simulink model "DVA_P1"  (R2020a)
settings: Solver=VariableStepAuto  StartTime=0.0  StopTime=10.0  MaxStep=0.001  RelTol=1e-3
settings Model: Creator=DELL  LastModifiedBy=DELL

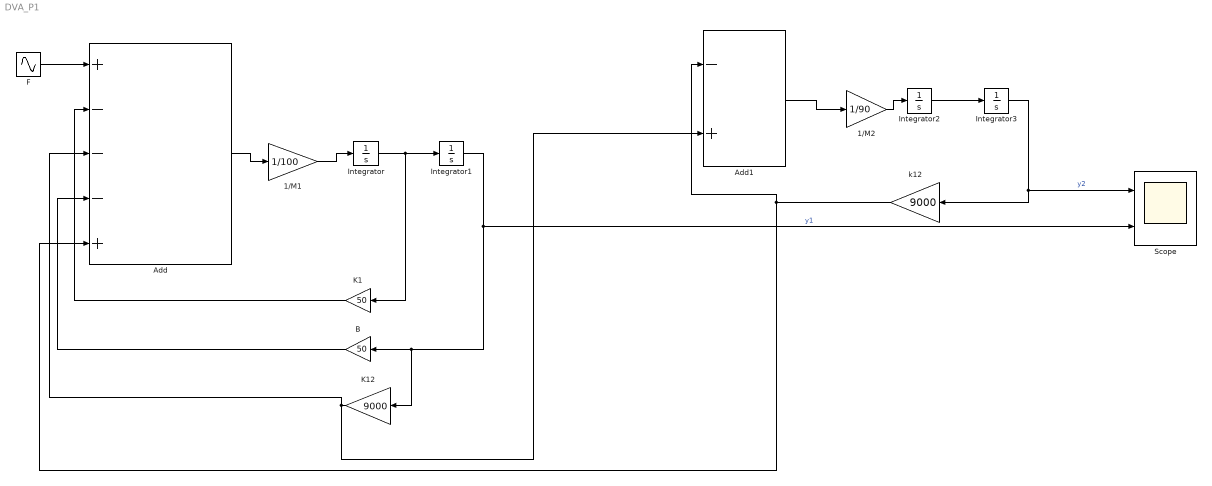
== system DVA_P1 ==
  1/M1 : Gain  Gain=1/100
  1/M2 : Gain  Gain=1/90
  Add : Sum  Inputs=+---+
  Add1 : Sum  Inputs=-+
  B : Gain  Gain=50
  F : Sin  Amplitude=2  Frequency=10  SampleTime=0
  Integrator{,1..3} (4 alike) : Integrator
  K1 : Gain  Gain=50
  K12 : Gain  Gain=9000
  Scope : Scope  NumInputPorts=2
  k12 : Gain  Gain=9000
  wires:
  Add/1 -> 1/M1/1
  Integrator/1 -> K1/1, Integrator1/1
  1/M1/1 -> Integrator/1
  Integrator1/1 -> Scope/2, K12/1, B/1  "y1"
  F/1 -> Add/1
  K1/1 -> Add/2
  B/1 -> Add/4
  K12/1 -> Add/3, Add1/2
  k12/1 -> Add1/1, Add/5
  Add1/1 -> 1/M2/1
  Integrator3/1 -> k12/1, Scope/1  "y2"
  1/M2/1 -> Integrator2/1
  Integrator2/1 -> Integrator3/1
